simulink model "Model_with_decision_and_sieve"  (R2022a)
settings: Solver=VariableStepAuto  StartTime=0.0  StopTime=1000000  RelTol=1e-3
undefined symbols (not defined in the file): Coefficient_value, Enable_X, Enable_Y, N, s1, s10, s11, s12, s13, s14, s15, s16, s17, s18, s19, s2, s20, s21, s22, s23, s24, s25, s26, s27, s28, s29, s3, s30, s4, s5, s6, s7, s8, s9
libraries: simulink x37, dspsigops x2
(part 5 of 5)

== system Model_with_decision_and_sieve/Pbit_2/EN=1 Block ==
  note: this is boolean
  note: threshold is subtracted from the sum of total input and random value to implement > 1 comparison
  IN : Inport
  Action Port : ActionPort  ActionPortLabel=if(u1 > 0)
  Add : Sum
  Add1 : Sum
  Compare To Constant : simulink/Logic and Bit Operations/Compare To Constant  relop=>  const=1  OutDataTypeStr=boolean
  Constant : Constant  Value=-1
  Constant1 : Constant
  Constant2 : Constant
  Divide : Product  Inputs=*/
  Math Function : Math
  Product : Product
  Uniform Random Number : UniformRandomNumber  Minimum=0  Seed=s2  SampleTime=1
  OUT : Outport
  wires:
  Add1/1 -> Divide/2
  Constant2/1 -> Divide/1
  Math Function/1 -> Add1/1
  Product/1 -> Math Function/1
  Constant1/1 -> Add1/2
  Constant/1 -> Product/2
  Divide/1 -> Add/1
  IN/1 -> Product/1
  Compare To Constant/1 -> OUT/1
  Add/1 -> Compare To Constant/1
  Uniform Random Number/1 -> Add/2

== system Model_with_decision_and_sieve/Pbit_3/EN=0 Block ==
  IN : Inport
  Action Port : ActionPort  ActionPortLabel=else
  Out1 : Outport
  wires:
  IN/1 -> Out1/1

== system Model_with_decision_and_sieve/Pbit_3/EN=1 Block ==
  note: threshold is subtracted from the sum of total input and random value to implement > 1 comparison
  note: this is boolean
  IN : Inport
  Action Port : ActionPort  ActionPortLabel=if(u1 > 0)
  Add : Sum
  Add1 : Sum
  Compare To Constant : simulink/Logic and Bit Operations/Compare To Constant  relop=>  const=1  OutDataTypeStr=boolean
  Constant : Constant  Value=-1
  Constant1 : Constant
  Constant2 : Constant
  Divide : Product  Inputs=*/
  Math Function : Math
  Product : Product
  Uniform Random Number : UniformRandomNumber  Minimum=0  Seed=s3  SampleTime=1
  OUT : Outport
  wires:
  Uniform Random Number/1 -> Add/2
  Add/1 -> Compare To Constant/1
  Compare To Constant/1 -> OUT/1
  IN/1 -> Product/1
  Divide/1 -> Add/1
  Constant/1 -> Product/2
  Constant1/1 -> Add1/2
  Product/1 -> Math Function/1
  Math Function/1 -> Add1/1
  Constant2/1 -> Divide/1
  Add1/1 -> Divide/2

== system Model_with_decision_and_sieve/Pbit_4/EN=0 Block ==
  IN : Inport
  Action Port : ActionPort  ActionPortLabel=else
  Out1 : Outport
  wires:
  IN/1 -> Out1/1

== system Model_with_decision_and_sieve/Pbit_4/EN=1 Block ==
  note: threshold is subtracted from the sum of total input and random value to implement > 1 comparison
  note: this is boolean
  IN : Inport
  Action Port : ActionPort  ActionPortLabel=if(u1 > 0)
  Add : Sum
  Add1 : Sum
  Compare To Constant : simulink/Logic and Bit Operations/Compare To Constant  relop=>  const=1  OutDataTypeStr=boolean
  Constant : Constant  Value=-1
  Constant1 : Constant
  Constant2 : Constant
  Divide : Product  Inputs=*/
  Math Function : Math
  Product : Product
  Uniform Random Number : UniformRandomNumber  Minimum=0  Seed=s4  SampleTime=1
  OUT : Outport
  wires:
  Uniform Random Number/1 -> Add/2
  Add/1 -> Compare To Constant/1
  Compare To Constant/1 -> OUT/1
  IN/1 -> Product/1
  Divide/1 -> Add/1
  Constant/1 -> Product/2
  Constant1/1 -> Add1/2
  Product/1 -> Math Function/1
  Math Function/1 -> Add1/1
  Constant2/1 -> Divide/1
  Add1/1 -> Divide/2

== system Model_with_decision_and_sieve/Pbit_5/EN=0 Block ==
  IN : Inport
  Action Port : ActionPort  ActionPortLabel=else
  Out1 : Outport
  wires:
  IN/1 -> Out1/1

== system Model_with_decision_and_sieve/Pbit_5/EN=1 Block ==
  note: this is boolean
  note: threshold is subtracted from the sum of total input and random value to implement > 1 comparison
  IN : Inport
  Action Port : ActionPort  ActionPortLabel=if(u1 > 0)
  Add : Sum
  Add1 : Sum
  Compare To Constant : simulink/Logic and Bit Operations/Compare To Constant  relop=>  const=1  OutDataTypeStr=boolean
  Constant : Constant  Value=-1
  Constant1 : Constant
  Constant2 : Constant
  Divide : Product  Inputs=*/
  Math Function : Math
  Product : Product
  Uniform Random Number : UniformRandomNumber  Minimum=0  Seed=s5  SampleTime=1
  OUT : Outport
  wires:
  Add1/1 -> Divide/2
  Constant2/1 -> Divide/1
  Math Function/1 -> Add1/1
  Product/1 -> Math Function/1
  Constant1/1 -> Add1/2
  Constant/1 -> Product/2
  Divide/1 -> Add/1
  IN/1 -> Product/1
  Compare To Constant/1 -> OUT/1
  Add/1 -> Compare To Constant/1
  Uniform Random Number/1 -> Add/2

== system Model_with_decision_and_sieve/Pbit_6/EN=0 Block ==
  IN : Inport
  Action Port : ActionPort  ActionPortLabel=else
  Out1 : Outport
  wires:
  IN/1 -> Out1/1

== system Model_with_decision_and_sieve/Pbit_6/EN=1 Block ==
  note: this is boolean
  note: threshold is subtracted from the sum of total input and random value to implement > 1 comparison
  IN : Inport
  Action Port : ActionPort  ActionPortLabel=if(u1 > 0)
  Add : Sum
  Add1 : Sum
  Compare To Constant : simulink/Logic and Bit Operations/Compare To Constant  relop=>  const=1  OutDataTypeStr=boolean
  Constant : Constant  Value=-1
  Constant1 : Constant
  Constant2 : Constant
  Divide : Product  Inputs=*/
  Math Function : Math
  Product : Product
  Uniform Random Number : UniformRandomNumber  Minimum=0  Seed=s6  SampleTime=1
  OUT : Outport
  wires:
  Add1/1 -> Divide/2
  Constant2/1 -> Divide/1
  Math Function/1 -> Add1/1
  Product/1 -> Math Function/1
  Constant1/1 -> Add1/2
  Constant/1 -> Product/2
  Divide/1 -> Add/1
  IN/1 -> Product/1
  Compare To Constant/1 -> OUT/1
  Add/1 -> Compare To Constant/1
  Uniform Random Number/1 -> Add/2

== system Model_with_decision_and_sieve/Pbit_7/EN=0 Block ==
  IN : Inport
  Action Port : ActionPort  ActionPortLabel=else
  Out1 : Outport
  wires:
  IN/1 -> Out1/1

== system Model_with_decision_and_sieve/Pbit_7/EN=1 Block ==
  note: this is boolean
  note: threshold is subtracted from the sum of total input and random value to implement > 1 comparison
  IN : Inport
  Action Port : ActionPort  ActionPortLabel=if(u1 > 0)
  Add : Sum
  Add1 : Sum
  Compare To Constant : simulink/Logic and Bit Operations/Compare To Constant  relop=>  const=1  OutDataTypeStr=boolean
  Constant : Constant  Value=-1
  Constant1 : Constant
  Constant2 : Constant
  Divide : Product  Inputs=*/
  Math Function : Math
  Product : Product
  Uniform Random Number : UniformRandomNumber  Minimum=0  Seed=s7  SampleTime=1
  OUT : Outport
  wires:
  Add1/1 -> Divide/2
  Constant2/1 -> Divide/1
  Math Function/1 -> Add1/1
  Product/1 -> Math Function/1
  Constant1/1 -> Add1/2
  Constant/1 -> Product/2
  Divide/1 -> Add/1
  IN/1 -> Product/1
  Compare To Constant/1 -> OUT/1
  Add/1 -> Compare To Constant/1
  Uniform Random Number/1 -> Add/2

== system Model_with_decision_and_sieve/Pbit_8/EN=0 Block ==
  IN : Inport
  Action Port : ActionPort  ActionPortLabel=else
  Out1 : Outport
  wires:
  IN/1 -> Out1/1

== system Model_with_decision_and_sieve/Pbit_8/EN=1 Block ==
  note: threshold is subtracted from the sum of total input and random value to implement > 1 comparison
  note: this is boolean
  IN : Inport
  Action Port : ActionPort  ActionPortLabel=if(u1 > 0)
  Add : Sum
  Add1 : Sum
  Compare To Constant : simulink/Logic and Bit Operations/Compare To Constant  relop=>  const=1  OutDataTypeStr=boolean
  Constant : Constant  Value=-1
  Constant1 : Constant
  Constant2 : Constant
  Divide : Product  Inputs=*/
  Math Function : Math
  Product : Product
  Uniform Random Number : UniformRandomNumber  Minimum=0  Seed=s8  SampleTime=1
  OUT : Outport
  wires:
  Uniform Random Number/1 -> Add/2
  Add/1 -> Compare To Constant/1
  Compare To Constant/1 -> OUT/1
  IN/1 -> Product/1
  Divide/1 -> Add/1
  Constant/1 -> Product/2
  Constant1/1 -> Add1/2
  Product/1 -> Math Function/1
  Math Function/1 -> Add1/1
  Constant2/1 -> Divide/1
  Add1/1 -> Divide/2

== system Model_with_decision_and_sieve/Pbit_9/EN=0 Block ==
  IN : Inport
  Action Port : ActionPort  ActionPortLabel=else
  Out1 : Outport
  wires:
  IN/1 -> Out1/1

== system Model_with_decision_and_sieve/Pbit_9/EN=1 Block ==
  note: threshold is subtracted from the sum of total input and random value to implement > 1 comparison
  note: this is boolean
  IN : Inport
  Action Port : ActionPort  ActionPortLabel=if(u1 > 0)
  Add : Sum
  Add1 : Sum
  Compare To Constant : simulink/Logic and Bit Operations/Compare To Constant  relop=>  const=1  OutDataTypeStr=boolean
  Constant : Constant  Value=-1
  Constant1 : Constant
  Constant2 : Constant
  Divide : Product  Inputs=*/
  Math Function : Math
  Product : Product
  Uniform Random Number : UniformRandomNumber  Minimum=0  Seed=s9  SampleTime=1
  OUT : Outport
  wires:
  Uniform Random Number/1 -> Add/2
  Add/1 -> Compare To Constant/1
  Compare To Constant/1 -> OUT/1
  IN/1 -> Product/1
  Divide/1 -> Add/1
  Constant/1 -> Product/2
  Constant1/1 -> Add1/2
  Product/1 -> Math Function/1
  Math Function/1 -> Add1/1
  Constant2/1 -> Divide/1
  Add1/1 -> Divide/2

== system Model_with_decision_and_sieve/Pbit_Y_1/EN=0 Block ==
  IN : Inport
  Action Port : ActionPort  ActionPortLabel=else
  Out1 : Outport
  wires:
  IN/1 -> Out1/1

== system Model_with_decision_and_sieve/Pbit_Y_1/EN=1 Block ==
  note: this is boolean
  note: threshold is subtracted from the sum of total input and random value to implement > 1 comparison
  IN : Inport
  Action Port : ActionPort  ActionPortLabel=if(u1 > 0)
  Add : Sum
  Add1 : Sum
  Compare To Constant : simulink/Logic and Bit Operations/Compare To Constant  relop=>  const=1  OutDataTypeStr=boolean
  Constant : Constant  Value=-1
  Constant1 : Constant
  Constant2 : Constant
  Divide : Product  Inputs=*/
  Math Function : Math
  Product : Product
  Uniform Random Number : UniformRandomNumber  Minimum=0  Seed=s16  SampleTime=1
  OUT : Outport
  wires:
  Add1/1 -> Divide/2
  Constant2/1 -> Divide/1
  Math Function/1 -> Add1/1
  Product/1 -> Math Function/1
  Constant1/1 -> Add1/2
  Constant/1 -> Product/2
  Divide/1 -> Add/1
  IN/1 -> Product/1
  Compare To Constant/1 -> OUT/1
  Add/1 -> Compare To Constant/1
  Uniform Random Number/1 -> Add/2

== system Model_with_decision_and_sieve/Pbit_Y_10/EN=0 Block ==
  IN : Inport
  Action Port : ActionPort  ActionPortLabel=else
  Out1 : Outport
  wires:
  IN/1 -> Out1/1

== system Model_with_decision_and_sieve/Pbit_Y_10/EN=1 Block ==
  note: this is boolean
  note: threshold is subtracted from the sum of total input and random value to implement > 1 comparison
  IN : Inport
  Action Port : ActionPort  ActionPortLabel=if(u1 > 0)
  Add : Sum
  Add1 : Sum
  Compare To Constant : simulink/Logic and Bit Operations/Compare To Constant  relop=>  const=1  OutDataTypeStr=boolean
  Constant : Constant  Value=-1
  Constant1 : Constant
  Constant2 : Constant
  Divide : Product  Inputs=*/
  Math Function : Math
  Product : Product
  Uniform Random Number : UniformRandomNumber  Minimum=0  Seed=s25  SampleTime=1
  OUT : Outport
  wires:
  Add1/1 -> Divide/2
  Constant2/1 -> Divide/1
  Math Function/1 -> Add1/1
  Product/1 -> Math Function/1
  Constant1/1 -> Add1/2
  Constant/1 -> Product/2
  Divide/1 -> Add/1
  IN/1 -> Product/1
  Compare To Constant/1 -> OUT/1
  Add/1 -> Compare To Constant/1
  Uniform Random Number/1 -> Add/2

== system Model_with_decision_and_sieve/Pbit_Y_11/EN=0 Block ==
  IN : Inport
  Action Port : ActionPort  ActionPortLabel=else
  Out1 : Outport
  wires:
  IN/1 -> Out1/1

== system Model_with_decision_and_sieve/Pbit_Y_11/EN=1 Block ==
  note: this is boolean
  note: threshold is subtracted from the sum of total input and random value to implement > 1 comparison
  IN : Inport
  Action Port : ActionPort  ActionPortLabel=if(u1 > 0)
  Add : Sum
  Add1 : Sum
  Compare To Constant : simulink/Logic and Bit Operations/Compare To Constant  relop=>  const=1  OutDataTypeStr=boolean
  Constant : Constant  Value=-1
  Constant1 : Constant
  Constant2 : Constant
  Divide : Product  Inputs=*/
  Math Function : Math
  Product : Product
  Uniform Random Number : UniformRandomNumber  Minimum=0  Seed=s26  SampleTime=1
  OUT : Outport
  wires:
  Add1/1 -> Divide/2
  Constant2/1 -> Divide/1
  Math Function/1 -> Add1/1
  Product/1 -> Math Function/1
  Constant1/1 -> Add1/2
  Constant/1 -> Product/2
  Divide/1 -> Add/1
  IN/1 -> Product/1
  Compare To Constant/1 -> OUT/1
  Add/1 -> Compare To Constant/1
  Uniform Random Number/1 -> Add/2

== system Model_with_decision_and_sieve/Pbit_Y_12/EN=0 Block ==
  IN : Inport
  Action Port : ActionPort  ActionPortLabel=else
  Out1 : Outport
  wires:
  IN/1 -> Out1/1

== system Model_with_decision_and_sieve/Pbit_Y_12/EN=1 Block ==
  note: this is boolean
  note: threshold is subtracted from the sum of total input and random value to implement > 1 comparison
  IN : Inport
  Action Port : ActionPort  ActionPortLabel=if(u1 > 0)
  Add : Sum
  Add1 : Sum
  Compare To Constant : simulink/Logic and Bit Operations/Compare To Constant  relop=>  const=1  OutDataTypeStr=boolean
  Constant : Constant  Value=-1
  Constant1 : Constant
  Constant2 : Constant
  Divide : Product  Inputs=*/
  Math Function : Math
  Product : Product
  Uniform Random Number : UniformRandomNumber  Minimum=0  Seed=s27  SampleTime=1
  OUT : Outport
  wires:
  Add1/1 -> Divide/2
  Constant2/1 -> Divide/1
  Math Function/1 -> Add1/1
  Product/1 -> Math Function/1
  Constant1/1 -> Add1/2
  Constant/1 -> Product/2
  Divide/1 -> Add/1
  IN/1 -> Product/1
  Compare To Constant/1 -> OUT/1
  Add/1 -> Compare To Constant/1
  Uniform Random Number/1 -> Add/2

== system Model_with_decision_and_sieve/Pbit_Y_13/EN=0 Block ==
  IN : Inport
  Action Port : ActionPort  ActionPortLabel=else
  Out1 : Outport
  wires:
  IN/1 -> Out1/1

== system Model_with_decision_and_sieve/Pbit_Y_13/EN=1 Block ==
  note: threshold is subtracted from the sum of total input and random value to implement > 1 comparison
  note: this is boolean
  IN : Inport
  Action Port : ActionPort  ActionPortLabel=if(u1 > 0)
  Add : Sum
  Add1 : Sum
  Compare To Constant : simulink/Logic and Bit Operations/Compare To Constant  relop=>  const=1  OutDataTypeStr=boolean
  Constant : Constant  Value=-1
  Constant1 : Constant
  Constant2 : Constant
  Divide : Product  Inputs=*/
  Math Function : Math
  Product : Product
  Uniform Random Number : UniformRandomNumber  Minimum=0  Seed=s28  SampleTime=1
  OUT : Outport
  wires:
  Uniform Random Number/1 -> Add/2
  Add/1 -> Compare To Constant/1
  Compare To Constant/1 -> OUT/1
  IN/1 -> Product/1
  Divide/1 -> Add/1
  Constant/1 -> Product/2
  Constant1/1 -> Add1/2
  Product/1 -> Math Function/1
  Math Function/1 -> Add1/1
  Constant2/1 -> Divide/1
  Add1/1 -> Divide/2

== system Model_with_decision_and_sieve/Pbit_Y_14/EN=0 Block ==
  IN : Inport
  Action Port : ActionPort  ActionPortLabel=else
  Out1 : Outport
  wires:
  IN/1 -> Out1/1

== system Model_with_decision_and_sieve/Pbit_Y_14/EN=1 Block ==
  note: threshold is subtracted from the sum of total input and random value to implement > 1 comparison
  note: this is boolean
  IN : Inport
  Action Port : ActionPort  ActionPortLabel=if(u1 > 0)
  Add : Sum
  Add1 : Sum
  Compare To Constant : simulink/Logic and Bit Operations/Compare To Constant  relop=>  const=1  OutDataTypeStr=boolean
  Constant : Constant  Value=-1
  Constant1 : Constant
  Constant2 : Constant
  Divide : Product  Inputs=*/
  Math Function : Math
  Product : Product
  Uniform Random Number : UniformRandomNumber  Minimum=0  Seed=s29  SampleTime=1
  OUT : Outport
  wires:
  Uniform Random Number/1 -> Add/2
  Add/1 -> Compare To Constant/1
  Compare To Constant/1 -> OUT/1
  IN/1 -> Product/1
  Divide/1 -> Add/1
  Constant/1 -> Product/2
  Constant1/1 -> Add1/2
  Product/1 -> Math Function/1
  Math Function/1 -> Add1/1
  Constant2/1 -> Divide/1
  Add1/1 -> Divide/2

== system Model_with_decision_and_sieve/Pbit_Y_15/EN=0 Block ==
  IN : Inport
  Action Port : ActionPort  ActionPortLabel=else
  Out1 : Outport
  wires:
  IN/1 -> Out1/1

== system Model_with_decision_and_sieve/Pbit_Y_15/EN=1 Block ==
  note: threshold is subtracted from the sum of total input and random value to implement > 1 comparison
  note: this is boolean
  IN : Inport
  Action Port : ActionPort  ActionPortLabel=if(u1 > 0)
  Add : Sum
  Add1 : Sum
  Compare To Constant : simulink/Logic and Bit Operations/Compare To Constant  relop=>  const=1  OutDataTypeStr=boolean
  Constant : Constant  Value=-1
  Constant1 : Constant
  Constant2 : Constant
  Divide : Product  Inputs=*/
  Math Function : Math
  Product : Product
  Uniform Random Number : UniformRandomNumber  Minimum=0  Seed=s30  SampleTime=1
  OUT : Outport
  wires:
  Uniform Random Number/1 -> Add/2
  Add/1 -> Compare To Constant/1
  Compare To Constant/1 -> OUT/1
  IN/1 -> Product/1
  Divide/1 -> Add/1
  Constant/1 -> Product/2
  Constant1/1 -> Add1/2
  Product/1 -> Math Function/1
  Math Function/1 -> Add1/1
  Constant2/1 -> Divide/1
  Add1/1 -> Divide/2

== system Model_with_decision_and_sieve/Pbit_Y_2/EN=0 Block ==
  IN : Inport
  Action Port : ActionPort  ActionPortLabel=else
  Out1 : Outport
  wires:
  IN/1 -> Out1/1

== system Model_with_decision_and_sieve/Pbit_Y_2/EN=1 Block ==
  note: this is boolean
  note: threshold is subtracted from the sum of total input and random value to implement > 1 comparison
  IN : Inport
  Action Port : ActionPort  ActionPortLabel=if(u1 > 0)
  Add : Sum
  Add1 : Sum
  Compare To Constant : simulink/Logic and Bit Operations/Compare To Constant  relop=>  const=1  OutDataTypeStr=boolean
  Constant : Constant  Value=-1
  Constant1 : Constant
  Constant2 : Constant
  Divide : Product  Inputs=*/
  Math Function : Math
  Product : Product
  Uniform Random Number : UniformRandomNumber  Minimum=0  Seed=s17  SampleTime=1
  OUT : Outport
  wires:
  Add1/1 -> Divide/2
  Constant2/1 -> Divide/1
  Math Function/1 -> Add1/1
  Product/1 -> Math Function/1
  Constant1/1 -> Add1/2
  Constant/1 -> Product/2
  Divide/1 -> Add/1
  IN/1 -> Product/1
  Compare To Constant/1 -> OUT/1
  Add/1 -> Compare To Constant/1
  Uniform Random Number/1 -> Add/2

== system Model_with_decision_and_sieve/Pbit_Y_3/EN=0 Block ==
  IN : Inport
  Action Port : ActionPort  ActionPortLabel=else
  Out1 : Outport
  wires:
  IN/1 -> Out1/1

== system Model_with_decision_and_sieve/Pbit_Y_3/EN=1 Block ==
  note: threshold is subtracted from the sum of total input and random value to implement > 1 comparison
  note: this is boolean
  IN : Inport
  Action Port : ActionPort  ActionPortLabel=if(u1 > 0)
  Add : Sum
  Add1 : Sum
  Compare To Constant : simulink/Logic and Bit Operations/Compare To Constant  relop=>  const=1  OutDataTypeStr=boolean
  Constant : Constant  Value=-1
  Constant1 : Constant
  Constant2 : Constant
  Divide : Product  Inputs=*/
  Math Function : Math
  Product : Product
  Uniform Random Number : UniformRandomNumber  Minimum=0  Seed=s18  SampleTime=1
  OUT : Outport
  wires:
  Uniform Random Number/1 -> Add/2
  Add/1 -> Compare To Constant/1
  Compare To Constant/1 -> OUT/1
  IN/1 -> Product/1
  Divide/1 -> Add/1
  Constant/1 -> Product/2
  Constant1/1 -> Add1/2
  Product/1 -> Math Function/1
  Math Function/1 -> Add1/1
  Constant2/1 -> Divide/1
  Add1/1 -> Divide/2

== system Model_with_decision_and_sieve/Pbit_Y_4/EN=0 Block ==
  IN : Inport
  Action Port : ActionPort  ActionPortLabel=else
  Out1 : Outport
  wires:
  IN/1 -> Out1/1

== system Model_with_decision_and_sieve/Pbit_Y_4/EN=1 Block ==
  note: threshold is subtracted from the sum of total input and random value to implement > 1 comparison
  note: this is boolean
  IN : Inport
  Action Port : ActionPort  ActionPortLabel=if(u1 > 0)
  Add : Sum
  Add1 : Sum
  Compare To Constant : simulink/Logic and Bit Operations/Compare To Constant  relop=>  const=1  OutDataTypeStr=boolean
  Constant : Constant  Value=-1
  Constant1 : Constant
  Constant2 : Constant
  Divide : Product  Inputs=*/
  Math Function : Math
  Product : Product
  Uniform Random Number : UniformRandomNumber  Minimum=0  Seed=s19  SampleTime=1
  OUT : Outport
  wires:
  Uniform Random Number/1 -> Add/2
  Add/1 -> Compare To Constant/1
  Compare To Constant/1 -> OUT/1
  IN/1 -> Product/1
  Divide/1 -> Add/1
  Constant/1 -> Product/2
  Constant1/1 -> Add1/2
  Product/1 -> Math Function/1
  Math Function/1 -> Add1/1
  Constant2/1 -> Divide/1
  Add1/1 -> Divide/2

== system Model_with_decision_and_sieve/Pbit_Y_5/EN=0 Block ==
  IN : Inport
  Action Port : ActionPort  ActionPortLabel=else
  Out1 : Outport
  wires:
  IN/1 -> Out1/1

== system Model_with_decision_and_sieve/Pbit_Y_5/EN=1 Block ==
  note: this is boolean
  note: threshold is subtracted from the sum of total input and random value to implement > 1 comparison
  IN : Inport
  Action Port : ActionPort  ActionPortLabel=if(u1 > 0)
  Add : Sum
  Add1 : Sum
  Compare To Constant : simulink/Logic and Bit Operations/Compare To Constant  relop=>  const=1  OutDataTypeStr=boolean
  Constant : Constant  Value=-1
  Constant1 : Constant
  Constant2 : Constant
  Divide : Product  Inputs=*/
  Math Function : Math
  Product : Product
  Uniform Random Number : UniformRandomNumber  Minimum=0  Seed=s20  SampleTime=1
  OUT : Outport
  wires:
  Add1/1 -> Divide/2
  Constant2/1 -> Divide/1
  Math Function/1 -> Add1/1
  Product/1 -> Math Function/1
  Constant1/1 -> Add1/2
  Constant/1 -> Product/2
  Divide/1 -> Add/1
  IN/1 -> Product/1
  Compare To Constant/1 -> OUT/1
  Add/1 -> Compare To Constant/1
  Uniform Random Number/1 -> Add/2

== system Model_with_decision_and_sieve/Pbit_Y_6/EN=0 Block ==
  IN : Inport
  Action Port : ActionPort  ActionPortLabel=else
  Out1 : Outport
  wires:
  IN/1 -> Out1/1

== system Model_with_decision_and_sieve/Pbit_Y_6/EN=1 Block ==
  note: this is boolean
  note: threshold is subtracted from the sum of total input and random value to implement > 1 comparison
  IN : Inport
  Action Port : ActionPort  ActionPortLabel=if(u1 > 0)
  Add : Sum
  Add1 : Sum
  Compare To Constant : simulink/Logic and Bit Operations/Compare To Constant  relop=>  const=1  OutDataTypeStr=boolean
  Constant : Constant  Value=-1
  Constant1 : Constant
  Constant2 : Constant
  Divide : Product  Inputs=*/
  Math Function : Math
  Product : Product
  Uniform Random Number : UniformRandomNumber  Minimum=0  Seed=s21  SampleTime=1
  OUT : Outport
  wires:
  Add1/1 -> Divide/2
  Constant2/1 -> Divide/1
  Math Function/1 -> Add1/1
  Product/1 -> Math Function/1
  Constant1/1 -> Add1/2
  Constant/1 -> Product/2
  Divide/1 -> Add/1
  IN/1 -> Product/1
  Compare To Constant/1 -> OUT/1
  Add/1 -> Compare To Constant/1
  Uniform Random Number/1 -> Add/2

== system Model_with_decision_and_sieve/Pbit_Y_7/EN=0 Block ==
  IN : Inport
  Action Port : ActionPort  ActionPortLabel=else
  Out1 : Outport
  wires:
  IN/1 -> Out1/1

== system Model_with_decision_and_sieve/Pbit_Y_7/EN=1 Block ==
  note: this is boolean
  note: threshold is subtracted from the sum of total input and random value to implement > 1 comparison
  IN : Inport
  Action Port : ActionPort  ActionPortLabel=if(u1 > 0)
  Add : Sum
  Add1 : Sum
  Compare To Constant : simulink/Logic and Bit Operations/Compare To Constant  relop=>  const=1  OutDataTypeStr=boolean
  Constant : Constant  Value=-1
  Constant1 : Constant
  Constant2 : Constant
  Divide : Product  Inputs=*/
  Math Function : Math
  Product : Product
  Uniform Random Number : UniformRandomNumber  Minimum=0  Seed=s22  SampleTime=1
  OUT : Outport
  wires:
  Add1/1 -> Divide/2
  Constant2/1 -> Divide/1
  Math Function/1 -> Add1/1
  Product/1 -> Math Function/1
  Constant1/1 -> Add1/2
  Constant/1 -> Product/2
  Divide/1 -> Add/1
  IN/1 -> Product/1
  Compare To Constant/1 -> OUT/1
  Add/1 -> Compare To Constant/1
  Uniform Random Number/1 -> Add/2

== system Model_with_decision_and_sieve/Pbit_Y_8/EN=0 Block ==
  IN : Inport
  Action Port : ActionPort  ActionPortLabel=else
  Out1 : Outport
  wires:
  IN/1 -> Out1/1

== system Model_with_decision_and_sieve/Pbit_Y_8/EN=1 Block ==
  note: threshold is subtracted from the sum of total input and random value to implement > 1 comparison
  note: this is boolean
  IN : Inport
  Action Port : ActionPort  ActionPortLabel=if(u1 > 0)
  Add : Sum
  Add1 : Sum
  Compare To Constant : simulink/Logic and Bit Operations/Compare To Constant  relop=>  const=1  OutDataTypeStr=boolean
  Constant : Constant  Value=-1
  Constant1 : Constant
  Constant2 : Constant
  Divide : Product  Inputs=*/
  Math Function : Math
  Product : Product
  Uniform Random Number : UniformRandomNumber  Minimum=0  Seed=s23  SampleTime=1
  OUT : Outport
  wires:
  Uniform Random Number/1 -> Add/2
  Add/1 -> Compare To Constant/1
  Compare To Constant/1 -> OUT/1
  IN/1 -> Product/1
  Divide/1 -> Add/1
  Constant/1 -> Product/2
  Constant1/1 -> Add1/2
  Product/1 -> Math Function/1
  Math Function/1 -> Add1/1
  Constant2/1 -> Divide/1
  Add1/1 -> Divide/2

== system Model_with_decision_and_sieve/Pbit_Y_9/EN=0 Block ==
  IN : Inport
  Action Port : ActionPort  ActionPortLabel=else
  Out1 : Outport
  wires:
  IN/1 -> Out1/1

== system Model_with_decision_and_sieve/Pbit_Y_9/EN=1 Block ==
  note: threshold is subtracted from the sum of total input and random value to implement > 1 comparison
  note: this is boolean
  IN : Inport
  Action Port : ActionPort  ActionPortLabel=if(u1 > 0)
  Add : Sum
  Add1 : Sum
  Compare To Constant : simulink/Logic and Bit Operations/Compare To Constant  relop=>  const=1  OutDataTypeStr=boolean
  Constant : Constant  Value=-1
  Constant1 : Constant
  Constant2 : Constant
  Divide : Product  Inputs=*/
  Math Function : Math
  Product : Product
  Uniform Random Number : UniformRandomNumber  Minimum=0  Seed=s24  SampleTime=1
  OUT : Outport
  wires:
  Uniform Random Number/1 -> Add/2
  Add/1 -> Compare To Constant/1
  Compare To Constant/1 -> OUT/1
  IN/1 -> Product/1
  Divide/1 -> Add/1
  Constant/1 -> Product/2
  Constant1/1 -> Add1/2
  Product/1 -> Math Function/1
  Math Function/1 -> Add1/1
  Constant2/1 -> Divide/1
  Add1/1 -> Divide/2

== system Model_with_decision_and_sieve/Sieve_X/Subsystem ==
  X : Inport
  Add : Sum
  Add1 : Sum  Inputs=+-
  Add2 : Sum
  Add3 : Sum  Inputs=+-
  Add4 : Sum  Inputs=+++++
  Constant{1,4,8,12,16} (5 alike) : Constant  Value=3
  Constant{3,6,10,14,18} (5 alike) : Constant  Value=7
  Constant11 : Constant  Value=2
  Constant{2,5,9,13,17} (5 alike) : Constant  Value=5
  Constant15 : Constant  Value=4
  Constant19 : Constant  Value=4
  Constant7 : Constant  Value=2
  Logical Operator : Logic  Inputs=3  AllPortsSameDT=off  OutDataTypeStr=boolean
  Logical Operator1 : Logic  Inputs=4  AllPortsSameDT=off  OutDataTypeStr=boolean
  Logical Operator{2..3,5,7} (4 alike) : Logic  Operator=NOT  Inputs=3  AllPortsSameDT=off  OutDataTypeStr=boolean
  Logical Operator4 : Logic  Inputs=5  AllPortsSameDT=off  OutDataTypeStr=boolean
  Logical Operator6 : Logic  Inputs=6  AllPortsSameDT=off  OutDataTypeStr=boolean
  Logical Operator8 : Logic  Inputs=7  AllPortsSameDT=off  OutDataTypeStr=boolean
  Mod{,1..14} (15 alike) : Math  Operator=mod  OutMax=1
  Product{,1..4} (5 alike) : Product
  Switch : Switch  Criteria=u2 ~= 0  SaturateOnIntegerOverflow=off  InputSameDT=off
  OUT : Outport
  wires:
  Mod/1 -> Logical Operator/1
  Constant2/1 -> Mod1/2
  Constant10/1 -> Mod8/2
  Mod2/1 -> Logical Operator/3
  Product1/1 -> Add4/2
  Add/1 -> Product1/1, Mod5/1, Mod4/1, Mod3/1
  Mod14/1 -> Logical Operator8/3
  Mod1/1 -> Logical Operator/2
  X/1 -> Add3/1, Add2/1, Add1/1, Add/1, Product/1, Mod2/1, Mod1/1, Mod/1
  Logical Operator1/1 -> Logical Operator3/1, Product1/2
  Add3/1 -> Switch/3, Product4/1, Mod14/1, Mod13/1, Mod12/1
  Constant11/1 -> Add1/2
  Constant3/1 -> Mod2/2
  Mod6/1 -> Logical Operator4/1
  Product4/1 -> Add4/5
  Add2/1 -> Product3/1, Mod11/1, Mod10/1, Mod9/1
  Constant16/1 -> Mod12/2
  Constant8/1 -> Mod6/2
  Mod10/1 -> Logical Operator6/2
  Add4/1 -> Switch/1, Switch/2
  Logical Operator7/1 -> Logical Operator8/7
  Mod7/1 -> Logical Operator4/2
  Mod9/1 -> Logical Operator6/1
  Constant19/1 -> Add3/2
  Mod8/1 -> Logical Operator4/3
  Switch/1 -> OUT/1
  Logical Operator/1 -> Logical Operator2/1, Product/2
  Logical Operator2/1 -> Logical Operator8/4, Logical Operator6/4, Logical Operator4/4, Logical Operator1/4
  Product3/1 -> Add4/4
  Logical Operator8/1 -> Product4/2
  Constant1/1 -> Mod/2
  Logical Operator4/1 -> Product2/2, Logical Operator5/1
  Constant5/1 -> Mod4/2
  Mod11/1 -> Logical Operator6/3
  Mod13/1 -> Logical Operator8/2
  Constant9/1 -> Mod7/2
  Mod4/1 -> Logical Operator1/2
  Constant18/1 -> Mod14/2
  Constant13/1 -> Mod10/2
  Logical Operator6/1 -> Product3/2, Logical Operator7/1
  Constant6/1 -> Mod5/2
  Product2/1 -> Add4/3
  Logical Operator5/1 -> Logical Operator8/6, Logical Operator6/6
  Logical Operator3/1 -> Logical Operator8/5, Logical Operator6/5, Logical Operator4/5
  Constant12/1 -> Mod9/2
  Constant15/1 -> Add2/2
  Mod12/1 -> Logical Operator8/1
  Constant14/1 -> Mod11/2
  Add1/1 -> Product2/1, Mod8/1, Mod7/1, Mod6/1
  Mod3/1 -> Logical Operator1/1
  Product/1 -> Add4/1
  Constant7/1 -> Add/2
  Mod5/1 -> Logical Operator1/3
  Constant17/1 -> Mod13/2
  Constant4/1 -> Mod3/2

== system Model_with_decision_and_sieve/Sieve_Y/Subsystem ==
  Y : Inport
  Add : Sum
  Add1 : Sum  Inputs=+-
  Add2 : Sum
  Add3 : Sum  Inputs=+-
  Add4 : Sum  Inputs=+++++
  Constant{1,4,8,12,16} (5 alike) : Constant  Value=3
  Constant{3,6,10,14,18} (5 alike) : Constant  Value=7
  Constant11 : Constant  Value=2
  Constant{2,5,9,13,17} (5 alike) : Constant  Value=5
  Constant15 : Constant  Value=4
  Constant19 : Constant  Value=4
  Constant7 : Constant  Value=2
  Logical Operator : Logic  Inputs=3  AllPortsSameDT=off  OutDataTypeStr=boolean
  Logical Operator1 : Logic  Inputs=4  AllPortsSameDT=off  OutDataTypeStr=boolean
  Logical Operator{2..3,5,7} (4 alike) : Logic  Operator=NOT  Inputs=3  AllPortsSameDT=off  OutDataTypeStr=boolean
  Logical Operator4 : Logic  Inputs=5  AllPortsSameDT=off  OutDataTypeStr=boolean
  Logical Operator6 : Logic  Inputs=6  AllPortsSameDT=off  OutDataTypeStr=boolean
  Logical Operator8 : Logic  Inputs=7  AllPortsSameDT=off  OutDataTypeStr=boolean
  Mod{,1..14} (15 alike) : Math  Operator=mod  OutMax=1
  Product{,1..4} (5 alike) : Product
  Switch : Switch  Criteria=u2 ~= 0  SaturateOnIntegerOverflow=off  InputSameDT=off
  OUT : Outport
  wires:
  Mod/1 -> Logical Operator/1
  Constant2/1 -> Mod1/2
  Constant10/1 -> Mod8/2
  Mod2/1 -> Logical Operator/3
  Product1/1 -> Add4/2
  Add/1 -> Product1/1, Mod5/1, Mod4/1, Mod3/1
  Mod14/1 -> Logical Operator8/3
  Mod1/1 -> Logical Operator/2
  Y/1 -> Add3/1, Add2/1, Add1/1, Add/1, Product/1, Mod2/1, Mod1/1, Mod/1
  Logical Operator1/1 -> Logical Operator3/1, Product1/2
  Add3/1 -> Switch/3, Product4/1, Mod14/1, Mod13/1, Mod12/1
  Constant11/1 -> Add1/2
  Constant3/1 -> Mod2/2
  Mod6/1 -> Logical Operator4/1
  Product4/1 -> Add4/5
  Add2/1 -> Product3/1, Mod11/1, Mod10/1, Mod9/1
  Constant16/1 -> Mod12/2
  Constant8/1 -> Mod6/2
  Mod10/1 -> Logical Operator6/2
  Add4/1 -> Switch/1, Switch/2
  Logical Operator7/1 -> Logical Operator8/7
  Mod7/1 -> Logical Operator4/2
  Mod9/1 -> Logical Operator6/1
  Constant19/1 -> Add3/2
  Mod8/1 -> Logical Operator4/3
  Switch/1 -> OUT/1
  Logical Operator/1 -> Logical Operator2/1, Product/2
  Logical Operator2/1 -> Logical Operator8/4, Logical Operator6/4, Logical Operator4/4, Logical Operator1/4
  Product3/1 -> Add4/4
  Logical Operator8/1 -> Product4/2
  Constant1/1 -> Mod/2
  Logical Operator4/1 -> Product2/2, Logical Operator5/1
  Constant5/1 -> Mod4/2
  Mod11/1 -> Logical Operator6/3
  Mod13/1 -> Logical Operator8/2
  Constant9/1 -> Mod7/2
  Mod4/1 -> Logical Operator1/2
  Constant18/1 -> Mod14/2
  Constant13/1 -> Mod10/2
  Logical Operator6/1 -> Product3/2, Logical Operator7/1
  Constant6/1 -> Mod5/2
  Product2/1 -> Add4/3
  Logical Operator5/1 -> Logical Operator8/6, Logical Operator6/6
  Logical Operator3/1 -> Logical Operator8/5, Logical Operator6/5, Logical Operator4/5
  Constant12/1 -> Mod9/2
  Constant15/1 -> Add2/2
  Mod12/1 -> Logical Operator8/1
  Constant14/1 -> Mod11/2
  Add1/1 -> Product2/1, Mod8/1, Mod7/1, Mod6/1
  Mod3/1 -> Logical Operator1/1
  Product/1 -> Add4/1
  Constant7/1 -> Add/2
  Mod5/1 -> Logical Operator1/3
  Constant17/1 -> Mod13/2
  Constant4/1 -> Mod3/2
